simulink model "pos_est_sil"  (R2024a)
settings: Solver=FixedStepAuto  StartTime=2  StopTime=615  FixedStep=0.002  RelTol=1e-3
libraries: simulink_extras x3
settings Model: PauseTimes=23.4  Creator=Zhenkai  LastModifiedBy=Zhenkai
settings DataIOCC: ReturnWorkspaceOutputs=off

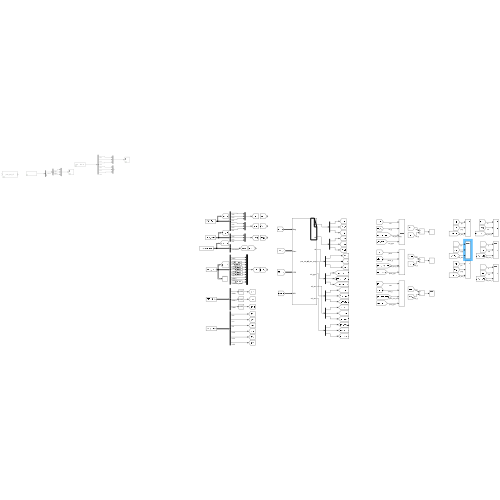
[thumbnail: Simulink's stored preview of the top-level diagram]
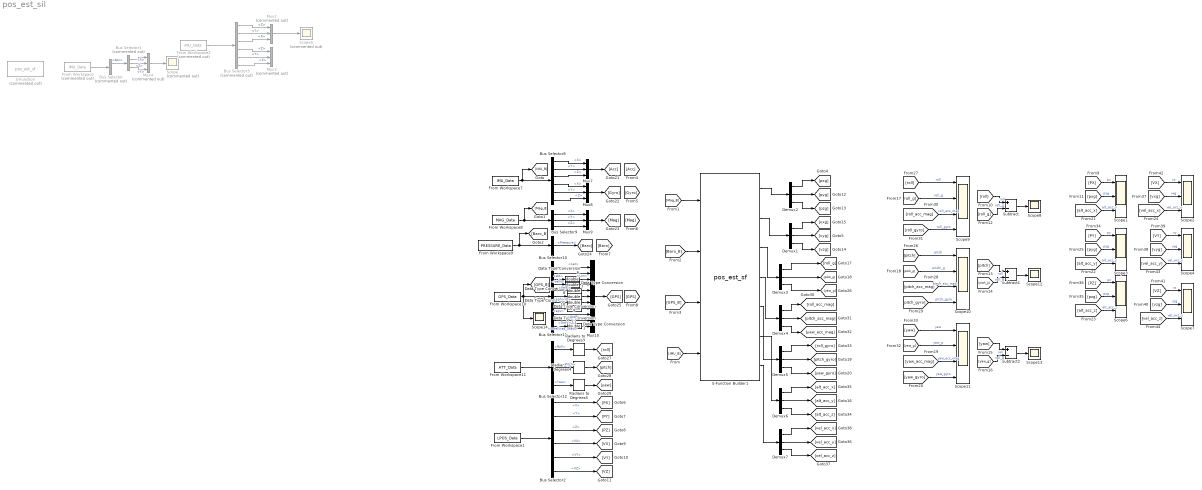
== system pos_est_sil ==
  Bus Selector : BusSelector  Commented=on  OutputSignals=Acc,Gyro
  Bus Selector1 : BusSelector  Commented=on  OutputSignals=X,Z,Y
  Bus Selector10 : BusSelector  OutputSignals=Pressure
  Bus Selector11 : BusSelector  OutputSignals=Lat,Lon,Alt,VelN,VelE,VelD,eph,epv,GotP,GotV,satellites_used
  Bus Selector12 : BusSelector  OutputSignals=Roll,Pitch,Yaw
  Bus Selector2 : BusSelector  OutputSignals=X,Y,Z,VX,VY,VZ
  Bus Selector3 : BusSelector  Commented=on  OutputSignals=Gyro.Z,Gyro.Y,Gyro.X,Acc.Z,Acc.Y,Acc.X
  Bus Selector8 : BusSelector  OutputSignals=Acc.X,Acc.Y,Acc.Z,Gyro.X,Gyro.Y,Gyro.Z
  Bus Selector9 : BusSelector  OutputSignals=X,Y,Z
  Data Type Conversion{1,6..11} (7 alike) : DataTypeConversion  OutDataTypeStr=double  SaturateOnIntegerOverflow=off  RndMeth=Floor
  Demux{1..7} (7 alike) : Demux  Outputs=3
  From Workspace : FromWorkspace  Commented=on  VariableName=IMU_Data  OutDataTypeStr=Bus: IMU_Bus  Interpolate=off  ZeroCross=off  OutputAfterFinalValue=Holding final value
  From Workspace1 : FromWorkspace  VariableName=LPOS_Data  OutDataTypeStr=Bus: LPOS_Bus
  From Workspace10 : FromWorkspace  VariableName=GPS_Data  OutDataTypeStr=Bus: GPS_Bus  Interpolate=off  OutputAfterFinalValue=Holding final value
  From Workspace11 : FromWorkspace  VariableName=ATT_Data  OutDataTypeStr=Bus: ATT_Bus
  From Workspace2 : FromWorkspace  Commented=on  VariableName=IMU_Data  OutDataTypeStr=Bus: IMU_Bus  Interpolate=off
  From Workspace7 : FromWorkspace  VariableName=IMU_Data  OutDataTypeStr=Bus: IMU_Bus  Interpolate=off  OutputAfterFinalValue=Holding final value
  From Workspace8 : FromWorkspace  VariableName=MAG_Data  OutDataTypeStr=Bus: MAG_Bus  Interpolate=off  OutputAfterFinalValue=Holding final value
  From Workspace9 : FromWorkspace  VariableName=PRESSURE_Data  OutDataTypeStr=Bus: PRESSURE_Bus  Interpolate=off  OutputAfterFinalValue=Holding final value
  Mux10 : Mux  Inputs=11
  Mux2 : Mux  Commented=on  Inputs=3
  Mux3 : Mux  Commented=on  Inputs=3
  Mux4 : Mux  Commented=on  Inputs=3
  Mux7 : Mux  Inputs=3
  Mux8 : Mux  Inputs=3
  Mux9 : Mux  Inputs=3
  Radians to Degrees3 : simulink_extras/Transformations/Radians to Degrees
  Radians to Degrees4 : simulink_extras/Transformations/Radians to Degrees
  Radians to Degrees5 : simulink_extras/Transformations/Radians to Degrees
  S-Function : S-Function  Commented=on  FunctionName=pos_est_sf  SFunctionDeploymentMode=off  EnableBusSupport=off
  S-Function Builder1 : S-Function  FunctionName=pos_est_sf  SFunctionModules=pos_est_sf_wrapper.c ringbuff com_data filter mahony attitude_estimate position_estimate task_integrated_navigation pro_common  SFunctionDeploymentMode=off  EnableBusSupport=off  mask(S-Function Builder){}
      mask help: Simulink:masks:SFunctionBuilder_MD
      mask init:
      | val = [[.9  0.75 0.75 1 1 .9 .9 1]',[1 1 0.75 0.75 .9 .9 1 .9]'];try , sys = get_param(gcb,'SfunBuilderFcnName');if isempty(sys), sys = get_param(gcb,'FunctionName'); end,catch, sys = get_param(gcb,'FunctionName'); end
      settings: CopyFcn=set_param(gcbh,'LinkStatus','none')  OpenFcn=sfunctionwizard(gcbh)
      mask Display:
      | plot(val(:,1),val(:,2))
      | disp(sys)
      | port_label('input',1,sprintf('%s', 'Mag'),'interpreter','tex')
      | port_label('input',2,sprintf('%s', 'Baro'),'interpreter','tex')
      | port_label('input',3,sprintf('%s', 'GPS'),'interpreter','tex')
      | port_label('input',4,sprintf('%s', 'IMU'),'interpreter','tex')
      | port_label('output',1,sprintf('%s', 'pos'),'interpreter','tex')
      | port_label('output',2,sprintf('%s', 'vel'),'interpreter','tex')
      | port_label('output',3,sprintf('%s', 'att'),'interpreter','tex')
      | port_label('output',4,sprintf('%s', 'att\_acc\_mag'),'interpreter','tex')
      | port_label('output',5,sprintf('%s', 'att\_gyro'),'interpreter','tex')
      | port_label('output',6,sprintf('%s', 'alt\_acc'),'interpreter','tex')
      | port_label('output',7,sprintf('%s', 'vel\_acc'),'interpreter','tex')
  Scope : Scope  Commented=on
  Scope{1..4,6..7} (6 alike) : Scope  NumInputPorts=3
  Scope10 : Scope  NumInputPorts=4
  Scope11 : Scope  NumInputPorts=4
  Scope{8,12..14} (4 alike) : Scope
  Scope5 : Scope  Commented=on
  Scope9 : Scope  NumInputPorts=4
  Subtract : Sum  Inputs=+-
  Subtract1 : Sum  Inputs=+-
  Subtract2 : Sum  Inputs=+-
  wires:
  From Workspace/1 -> Bus Selector/1
  Bus Selector/1 -> Bus Selector1/1  "<Acc>"
  Bus Selector3/2 -> Mux2/2  "<Y>"
  Bus Selector3/5 -> Mux3/2  "<Y>"
  Bus Selector3/3 -> Mux2/3  "<X>"
  Bus Selector3/6 -> Mux3/3  "<X>"
  From Workspace2/1 -> Bus Selector3/1
  Mux2/1 -> Scope5/1
  Bus Selector3/1 -> Mux2/1  "<Z>"
  Bus Selector3/4 -> Mux3/1  "<Z>"
  Bus Selector1/1 -> Mux4/1  "<X>"
  Bus Selector1/2 -> Mux4/2  "<Z>"
  Bus Selector1/3 -> Mux4/3  "<Y>"
  Mux4/1 -> Scope/1
  Bus Selector12/2 -> Radians to Degrees4/1  "<Pitch>"
  S-Function Builder1/5 -> Demux5/1
  Bus Selector8/4 -> Mux8/1  "<X>"
  Demux4/2 -> [pitch_acc_mag]
  Bus Selector12/1 -> Radians to Degrees3/1  "<Roll>"
  Demux4/1 -> [roll_acc_mag]
  [roll_acc_mag] -> Scope9/3  "roll_acc_mag"
  Mux10/1 -> [GPS]
  Bus Selector10/1 -> [Baro]  "<Pressure>"
  Data Type Conversion11/1 -> Mux10/8
  [roll] -> Scope9/1  "roll"
  [pitch_g] -> Scope10/2  "pitchl_g"
  Radians to Degrees5/1 -> [yaw]
  Mux9/1 -> [Mag]
  Bus Selector8/3 -> Mux7/3  "<Z>"
  Mux7/1 -> [Acc]
  Bus Selector11/5 -> Data Type Conversion8/1  "<VelE>"
  Demux4/3 -> [yaw_acc_mag]
  Bus Selector11/9 -> Mux10/9  "<GotP>"
  Radians to Degrees4/1 -> [pitch]
  [roll_gyro] -> Scope9/4  "roll_gyro"
  From Workspace11/1 -> Bus Selector12/1
  Demux3/1 -> [roll_g]
  [pitch_gyro] -> Scope10/4  "pitch_gyro"
  Demux5/1 -> [roll_gyro]
  Bus Selector12/3 -> Radians to Degrees5/1  "<Yaw>"
  [yaw] -> Scope11/1  "yaw"
  S-Function Builder1/3 -> Demux3/1
  Data Type Conversion10/1 -> Mux10/7
  Demux5/2 -> [pitch_gyro]
  Bus Selector11/2 -> Mux10/2  "<Lon>"
  From Workspace9/1 -> Bus Selector10/1, [Baro_B]
  Demux5/3 -> [yaw_gyro]
  Demux3/2 -> [pitch_g]
  Mux8/1 -> [Gyro]
  Demux3/3 -> [yaw_g]
  [yaw_gyro] -> Scope11/4  "yaw_gyro"
  [yaw_acc_mag] -> Scope11/3  "yaw_acc_mag"
  Data Type Conversion8/1 -> Mux10/5
  [yaw_g] -> Scope11/2  "yaw_g"
  Bus Selector9/2 -> Mux9/2  "<Y>"
  S-Function Builder1/1 -> Demux2/1
  [pitch] -> Scope10/1  "pitch"
  From Workspace7/1 -> [IMU_B], Bus Selector8/1
  Bus Selector11/6 -> Data Type Conversion9/1  "<VelD>"
  Bus Selector11/4 -> Data Type Conversion7/1  "<VelN>"
  Bus Selector9/3 -> Mux9/3  "<Z>"
  From Workspace8/1 -> [Mag_B], Bus Selector9/1
  Bus Selector11/1 -> Mux10/1  "<Lat>"
  Bus Selector8/6 -> Mux8/3  "<Z>"
  [roll_g] -> Scope9/2  "roll_g"
  Bus Selector11/3 -> Data Type Conversion6/1  "<Alt>"
  Bus Selector9/1 -> Mux9/1  "<X>"
  From Workspace10/1 -> Scope14/1, [GPS_B], Bus Selector11/1
  Data Type Conversion9/1 -> Mux10/6
  Radians to Degrees3/1 -> [roll]
  Bus Selector8/2 -> Mux7/2  "<Y>"
  S-Function Builder1/4 -> Demux4/1
  Data Type Conversion6/1 -> Mux10/3
  Bus Selector11/8 -> Data Type Conversion11/1  "<epv>"
  Bus Selector8/1 -> Mux7/1  "<X>"
  [pitch_acc_mag] -> Scope10/3  "pitch_acc_mag"
  Bus Selector11/7 -> Data Type Conversion10/1  "<eph>"
  Data Type Conversion7/1 -> Mux10/4
  Bus Selector8/5 -> Mux8/2  "<Y>"
  Bus Selector11/10 -> Mux10/10  "<GotV>"
  [Mag_B] -> S-Function Builder1/1
  [Baro_B] -> S-Function Builder1/2
  [GPS_B] -> S-Function Builder1/3
  [IMU_B] -> S-Function Builder1/4
  From Workspace1/1 -> Bus Selector2/1
  Bus Selector2/1 -> [PX]  "<X>"
  Bus Selector2/2 -> [PY]  "<Y>"
  Bus Selector2/3 -> [PZ]  "<Z>"
  Bus Selector2/6 -> [VZ]  "<VZ>"
  Bus Selector2/5 -> [VY]  "<VY>"
  Bus Selector2/4 -> [VX]  "<VX>"
  Demux2/1 -> [pxg]
  Demux2/2 -> [pyg]
  Demux2/3 -> [pzg]
  Demux1/3 -> [vzg]
  Demux1/2 -> [vyg]
  Demux1/1 -> [vxg]
  S-Function Builder1/2 -> Demux1/1
  [PX] -> Scope1/1  "px"
  [pxg] -> Scope1/2  "pxg"
  Bus Selector11/11 -> Data Type Conversion1/1  "<satellites_used>"
  Data Type Conversion1/1 -> Mux10/11
  Subtract/1 -> Scope8/1
  [roll_g] -> Subtract/2  "roll_g"
  [roll] -> Subtract/1  "roll"
  [pitch] -> Subtract1/1  "roll"
  [pitch_g] -> Subtract1/2  "roll_g"
  Subtract1/1 -> Scope12/1
  [yaw] -> Subtract2/1  "roll"
  [yaw_g] -> Subtract2/2  "roll_g"
  Subtract2/1 -> Scope13/1
  S-Function Builder1/6 -> Demux6/1
  Demux6/1 -> [alt_acc_x]
  Demux6/3 -> [alt_acc_z]
  Demux6/2 -> [alt_acc_y]
  S-Function Builder1/7 -> Demux7/1
  Demux7/1 -> [vel_acc_x]
  Demux7/3 -> [vel_acc_z]
  Demux7/2 -> [vel_acc_y]
  [alt_acc_x] -> Scope1/3  "alt_acc_x"
  [PY] -> Scope3/1  "py"
  [pyg] -> Scope3/2  "pyg"
  [alt_acc_y] -> Scope3/3  "alt_acc_y"
  [PZ] -> Scope6/1  "pz"
  [pzg] -> Scope6/2  "pzg"
  [alt_acc_z] -> Scope6/3  "alt_acc_z"
  [VX] -> Scope2/1  "vx"
  [vxg] -> Scope2/2  "vxg"
  [vel_acc_x] -> Scope2/3  "vel_acc_x"
  [VY] -> Scope4/1  "vy"
  [vyg] -> Scope4/2  "vyg"
  [vel_acc_y] -> Scope4/3  "vel_acc_x"
  [VZ] -> Scope7/1  "vz"
  [vzg] -> Scope7/2  "vzg"
  [vel_acc_z] -> Scope7/3  "vel_acc_x"
